simulink model "position_by_Adaptive_RBF_Attitude_by_supervised_RBFNN"  (R2015a)
settings: Solver=ode3  StartTime=0.0  StopTime=40  FixedStep=0.001  RelTol=1e-3
libraries: simulink x12, commnoisgen2 x5, dspsrcs4 x1
(part 1 of 2)
settings Model: SimulationMode=accelerator  Creator=user  LastModifiedBy=user

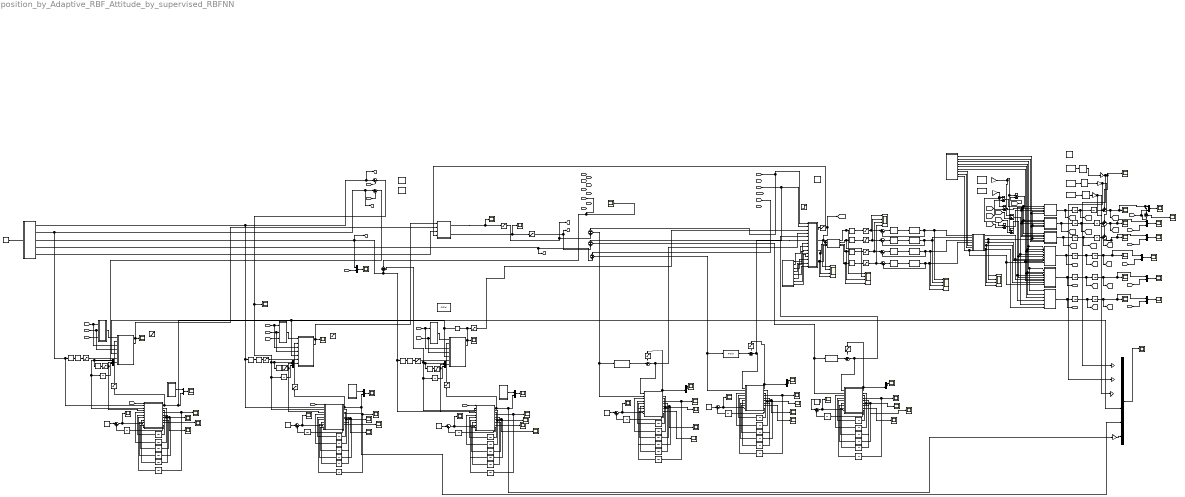
== system position_by_Adaptive_RBF_Attitude_by_supervised_RBFNN ==
  note: Linear position Adaptive RBF NN based control
  note: Attitude supervisory control based on RBF NN
  note: error of z
  note: 0.178
  note: 0.16
  note: used to extract data
  note: Adaptive RBFNN Position+ SUPERVISED RBF-PID attitude CONTROL-Final- VG results
  note: d25
  Constant{1..6} (6 alike) : Constant  Value=0
  DATA : MATLAB Function  TreatAsAtomicUnit=on
  DATA1 : MATLAB Function  TreatAsAtomicUnit=on
  Delay1 : Delay  DelayLength=1  SampleTime=0.001
  Derivative{,1..8} (9 alike) : Derivative
  Gain : Gain  Gain=0.01
  Gain1 : Gain  Gain=0.01
  Gain2 : Gain  Gain=2000
  Gain3 : Gain  Gain=2000
  Gain4 : Gain  Gain=2000
  Gain5 : Gain  Gain=0.1
  Gain6 : Gain  Gain=0.07
  Gain7 : Gain  Gain=0.07
  Gain8 : Gain  Gain=7
  Gaussian Noise Generator : commnoisgen2/Gaussian Noise Generator  m=0  d=1  s=41  Ts=0.02  frameBased=off  sampPerFrame=1  orient=off  outDataType=double
  Gaussian Noise Generator1 : commnoisgen2/Gaussian Noise Generator  m=0  d=1  s=41  Ts=0.02  frameBased=off  sampPerFrame=1  orient=off  outDataType=double
  Gaussian Noise Generator3 : commnoisgen2/Gaussian Noise Generator  m=0.3  d=1  s=41  Ts=5  frameBased=off  sampPerFrame=1  orient=off  outDataType=double
  Gaussian Noise Generator5 : commnoisgen2/Gaussian Noise Generator  m=0.3  d=1  s=41  Ts=2.5  frameBased=off  sampPerFrame=1  orient=off  outDataType=double
  Gaussian Noise Generator6 : commnoisgen2/Gaussian Noise Generator  m=0.3  d=1  s=41  Ts=3.5  frameBased=off  sampPerFrame=1  orient=on  outDataType=double
  Integrator{1..15} (15 alike) : Integrator
  MATLAB Function : MATLAB Function  TreatAsAtomicUnit=on
  MATLAB Function1 : MATLAB Function  TreatAsAtomicUnit=on
  MATLAB Function2 : MATLAB Function  TreatAsAtomicUnit=on
  MATLAB Function3 : MATLAB Function  TreatAsAtomicUnit=on
  MATLAB Function4 : MATLAB Function  TreatAsAtomicUnit=on
  MATLAB Function5 : MATLAB Function  TreatAsAtomicUnit=on
  MATLAB Function6 : MATLAB Function  TreatAsAtomicUnit=on
  MATLAB Function7 : MATLAB Function  TreatAsAtomicUnit=on
  MATLAB Function8 : MATLAB Function  TreatAsAtomicUnit=on
  Mux : Mux  Inputs=3
  Mux{1..10,12..13,15} (13 alike) : Mux  Inputs=2
  Mux11 : Mux  Inputs=3
  Mux14 : Mux  Inputs=3
  Mux16 : Mux  Inputs=6
  Omega i ^2  calc : MATLAB Function  TreatAsAtomicUnit=on
  Omegas : Scope  NumInputPorts=4
      settings: YMin=-5~-5~-5~-5  YMax=5~5~5~5  SaveName=ScopeData3
  PID Controller{,4..6} (4 alike) : simulink/Continuous/PID Controller  Controller=PID  TimeDomain=Continuous-time  SampleTime=-1  IntegratorMethod=Forward Euler  FilterMethod=Forward Euler  Form=Parallel  UseFilter=on  ControllerParametersSource=internal  P=0.696663945518539  I=69.3627675374527  D=0.000480635781112464  N=569.937710840054  InitialConditionSource=internal  InitialConditionForIntegrator=0  InitialConditionForFilter=0  ExternalReset=none  LimitOutput=off  UpperSaturationLimit=+12  LowerSaturationLimit=-12  LinearizeAsGain=on  AntiWindupMode=clamping  Kb=1  TrackingMode=off  Kt=1  PParamMin=[]  PParamMax=[]  IParamMin=[]  IParamMax=[]  DParamMin=[]  DParamMax=[]  NParamMin=[]  NParamMax=[]  KbParamMin=[]  KbParamMax=[]  KtParamMin=[]  KtParamMax=[]  POutMin=[]  POutMax=[]  IOutMin=[]  IOutMax=[]  DOutMin=[]  DOutMax=[]  NOutMin=[]  NOutMax=[]  KbOutMin=[]  KbOutMax=[]  KtOutMin=[]  KtOutMax=[]  IntegratorOutMin=[]  IntegratorOutMax=[]  FilterOutMin=[]  FilterOutMax=[]  SumOutMin=[]  SumOutMax=[]  SumI1OutMin=[]  SumI1OutMax=[]  SumI2OutMin=[]  SumI2OutMax=[]  SumI3OutMin=[]  SumI3OutMax=[]  SumDOutMin=[]  SumDOutMax=[]  SaturationOutMin=[]  SaturationOutMax=[]  IntegratorContinuousStateAttributes=''  IntegratorStateMustResolveToSignalObject=off  IntegratorRTWStateStorageClass=Auto  FilterContinuousStateAttributes=''  FilterStateMustResolveToSignalObject=off  FilterRTWStateStorageClass=Auto  DifferentiatorICPrevScaledInput=0  DifferentiatorOutMin=[]  DifferentiatorOutMax=[]
  PID Controller1 : simulink/Continuous/PID Controller  Controller=PID  TimeDomain=Continuous-time  SampleTime=-1  IntegratorMethod=Forward Euler  FilterMethod=Forward Euler  Form=Parallel  UseFilter=on  ControllerParametersSource=internal  P=4  I=2  D=5  N=476.409993785115  InitialConditionSource=internal  InitialConditionForIntegrator=0  InitialConditionForFilter=0  ExternalReset=none  LimitOutput=off  UpperSaturationLimit=inf  LowerSaturationLimit=-inf  LinearizeAsGain=on  AntiWindupMode=none  Kb=1  TrackingMode=off  Kt=1  PParamMin=[]  PParamMax=[]  IParamMin=[]  IParamMax=[]  DParamMin=[]  DParamMax=[]  NParamMin=[]  NParamMax=[]  KbParamMin=[]  KbParamMax=[]  KtParamMin=[]  KtParamMax=[]  POutMin=[]  POutMax=[]  IOutMin=[]  IOutMax=[]  DOutMin=[]  DOutMax=[]  NOutMin=[]  NOutMax=[]  KbOutMin=[]  KbOutMax=[]  KtOutMin=[]  KtOutMax=[]  IntegratorOutMin=[]  IntegratorOutMax=[]  FilterOutMin=[]  FilterOutMax=[]  SumOutMin=[]  SumOutMax=[]  SumI1OutMin=[]  SumI1OutMax=[]  SumI2OutMin=[]  SumI2OutMax=[]  SumI3OutMin=[]  SumI3OutMax=[]  SumDOutMin=[]  SumDOutMax=[]  SaturationOutMin=[]  SaturationOutMax=[]  IntegratorContinuousStateAttributes=''  IntegratorStateMustResolveToSignalObject=off  IntegratorRTWStateStorageClass=Auto  FilterContinuousStateAttributes=''  FilterStateMustResolveToSignalObject=off  FilterRTWStateStorageClass=Auto  DifferentiatorICPrevScaledInput=0  DifferentiatorOutMin=[]  DifferentiatorOutMax=[]
  PID Controller14 : simulink/Continuous/PID Controller  Controller=PID  TimeDomain=Continuous-time  SampleTime=-1  IntegratorMethod=Forward Euler  FilterMethod=Forward Euler  Form=Parallel  UseFilter=on  ControllerParametersSource=internal  P=1.8  I=0.4  D=2.4  N=100  InitialConditionSource=internal  InitialConditionForIntegrator=0  InitialConditionForFilter=0  ExternalReset=none  LimitOutput=off  UpperSaturationLimit=inf  LowerSaturationLimit=-inf  LinearizeAsGain=on  AntiWindupMode=none  Kb=1  TrackingMode=off  Kt=1  PParamMin=[]  PParamMax=[]  IParamMin=[]  IParamMax=[]  DParamMin=[]  DParamMax=[]  NParamMin=[]  NParamMax=[]  KbParamMin=[]  KbParamMax=[]  KtParamMin=[]  KtParamMax=[]  POutMin=[]  POutMax=[]  IOutMin=[]  IOutMax=[]  DOutMin=[]  DOutMax=[]  NOutMin=[]  NOutMax=[]  KbOutMin=[]  KbOutMax=[]  KtOutMin=[]  KtOutMax=[]  IntegratorOutMin=[]  IntegratorOutMax=[]  FilterOutMin=[]  FilterOutMax=[]  SumOutMin=[]  SumOutMax=[]  SumI1OutMin=[]  SumI1OutMax=[]  SumI2OutMin=[]  SumI2OutMax=[]  SumI3OutMin=[]  SumI3OutMax=[]  SumDOutMin=[]  SumDOutMax=[]  SaturationOutMin=[]  SaturationOutMax=[]  IntegratorContinuousStateAttributes=''  IntegratorStateMustResolveToSignalObject=off  IntegratorRTWStateStorageClass=Auto  FilterContinuousStateAttributes=''  FilterStateMustResolveToSignalObject=off  FilterRTWStateStorageClass=Auto  DifferentiatorICPrevScaledInput=0  DifferentiatorOutMin=[]  DifferentiatorOutMax=[]
  PID Controller15 : simulink/Continuous/PID Controller  Controller=PID  TimeDomain=Continuous-time  SampleTime=-1  IntegratorMethod=Forward Euler  FilterMethod=Forward Euler  Form=Parallel  UseFilter=on  ControllerParametersSource=internal  P=1.8  I=0.4  D=2.1  N=100  InitialConditionSource=internal  InitialConditionForIntegrator=0  InitialConditionForFilter=0  ExternalReset=none  LimitOutput=off  UpperSaturationLimit=inf  LowerSaturationLimit=-inf  LinearizeAsGain=on  AntiWindupMode=none  Kb=1  TrackingMode=off  Kt=1  PParamMin=[]  PParamMax=[]  IParamMin=[]  IParamMax=[]  DParamMin=[]  DParamMax=[]  NParamMin=[]  NParamMax=[]  KbParamMin=[]  KbParamMax=[]  KtParamMin=[]  KtParamMax=[]  POutMin=[]  POutMax=[]  IOutMin=[]  IOutMax=[]  DOutMin=[]  DOutMax=[]  NOutMin=[]  NOutMax=[]  KbOutMin=[]  KbOutMax=[]  KtOutMin=[]  KtOutMax=[]  IntegratorOutMin=[]  IntegratorOutMax=[]  FilterOutMin=[]  FilterOutMax=[]  SumOutMin=[]  SumOutMax=[]  SumI1OutMin=[]  SumI1OutMax=[]  SumI2OutMin=[]  SumI2OutMax=[]  SumI3OutMin=[]  SumI3OutMax=[]  SumDOutMin=[]  SumDOutMax=[]  SaturationOutMin=[]  SaturationOutMax=[]  IntegratorContinuousStateAttributes=''  IntegratorStateMustResolveToSignalObject=off  IntegratorRTWStateStorageClass=Auto  FilterContinuousStateAttributes=''  FilterStateMustResolveToSignalObject=off  FilterRTWStateStorageClass=Auto  DifferentiatorICPrevScaledInput=0  DifferentiatorOutMin=[]  DifferentiatorOutMax=[]
  PID Controller2 : simulink/Continuous/PID Controller  Controller=PID  TimeDomain=Continuous-time  SampleTime=-1  IntegratorMethod=Forward Euler  FilterMethod=Forward Euler  Form=Parallel  UseFilter=on  ControllerParametersSource=internal  P=4.05643234281984  I=0.70959032661118  D=4.0859309721323  N=476.409993785115  InitialConditionSource=internal  InitialConditionForIntegrator=0  InitialConditionForFilter=0  ExternalReset=none  LimitOutput=off  UpperSaturationLimit=inf  LowerSaturationLimit=-inf  LinearizeAsGain=on  AntiWindupMode=none  Kb=1  TrackingMode=off  Kt=1  PParamMin=[]  PParamMax=[]  IParamMin=[]  IParamMax=[]  DParamMin=[]  DParamMax=[]  NParamMin=[]  NParamMax=[]  KbParamMin=[]  KbParamMax=[]  KtParamMin=[]  KtParamMax=[]  POutMin=[]  POutMax=[]  IOutMin=[]  IOutMax=[]  DOutMin=[]  DOutMax=[]  NOutMin=[]  NOutMax=[]  KbOutMin=[]  KbOutMax=[]  KtOutMin=[]  KtOutMax=[]  IntegratorOutMin=[]  IntegratorOutMax=[]  FilterOutMin=[]  FilterOutMax=[]  SumOutMin=[]  SumOutMax=[]  SumI1OutMin=[]  SumI1OutMax=[]  SumI2OutMin=[]  SumI2OutMax=[]  SumI3OutMin=[]  SumI3OutMax=[]  SumDOutMin=[]  SumDOutMax=[]  SaturationOutMin=[]  SaturationOutMax=[]  IntegratorContinuousStateAttributes=''  IntegratorStateMustResolveToSignalObject=off  IntegratorRTWStateStorageClass=Auto  FilterContinuousStateAttributes=''  FilterStateMustResolveToSignalObject=off  FilterRTWStateStorageClass=Auto  DifferentiatorICPrevScaledInput=0  DifferentiatorOutMin=[]  DifferentiatorOutMax=[]
  PID Controller3 : simulink/Continuous/PID Controller  Controller=PID  TimeDomain=Continuous-time  SampleTime=-1  IntegratorMethod=Forward Euler  FilterMethod=Forward Euler  Form=Parallel  UseFilter=on  ControllerParametersSource=internal  P=11  I=0.2  D=22  N=100  InitialConditionSource=internal  InitialConditionForIntegrator=0  InitialConditionForFilter=0  ExternalReset=none  LimitOutput=off  UpperSaturationLimit=inf  LowerSaturationLimit=-inf  LinearizeAsGain=on  AntiWindupMode=none  Kb=1  TrackingMode=off  Kt=1  PParamMin=[]  PParamMax=[]  IParamMin=[]  IParamMax=[]  DParamMin=[]  DParamMax=[]  NParamMin=[]  NParamMax=[]  KbParamMin=[]  KbParamMax=[]  KtParamMin=[]  KtParamMax=[]  POutMin=[]  POutMax=[]  IOutMin=[]  IOutMax=[]  DOutMin=[]  DOutMax=[]  NOutMin=[]  NOutMax=[]  KbOutMin=[]  KbOutMax=[]  KtOutMin=[]  KtOutMax=[]  IntegratorOutMin=[]  IntegratorOutMax=[]  FilterOutMin=[]  FilterOutMax=[]  SumOutMin=[]  SumOutMax=[]  SumI1OutMin=[]  SumI1OutMax=[]  SumI2OutMin=[]  SumI2OutMax=[]  SumI3OutMin=[]  SumI3OutMax=[]  SumDOutMin=[]  SumDOutMax=[]  SaturationOutMin=[]  SaturationOutMax=[]  IntegratorContinuousStateAttributes=''  IntegratorStateMustResolveToSignalObject=off  IntegratorRTWStateStorageClass=Auto  FilterContinuousStateAttributes=''  FilterStateMustResolveToSignalObject=off  FilterRTWStateStorageClass=Auto  DifferentiatorICPrevScaledInput=0  DifferentiatorOutMin=[]  DifferentiatorOutMax=[]
  PID Controller7 : simulink/Continuous/PID Controller  Controller=PID  TimeDomain=Continuous-time  SampleTime=-1  IntegratorMethod=Forward Euler  FilterMethod=Forward Euler  Form=Parallel  UseFilter=on  ControllerParametersSource=internal  P=12  I=0.2  D=14  N=100  InitialConditionSource=internal  InitialConditionForIntegrator=0  InitialConditionForFilter=0  ExternalReset=none  LimitOutput=off  UpperSaturationLimit=inf  LowerSaturationLimit=-inf  LinearizeAsGain=on  AntiWindupMode=none  Kb=1  TrackingMode=off  Kt=1  PParamMin=[]  PParamMax=[]  IParamMin=[]  IParamMax=[]  DParamMin=[]  DParamMax=[]  NParamMin=[]  NParamMax=[]  KbParamMin=[]  KbParamMax=[]  KtParamMin=[]  KtParamMax=[]  POutMin=[]  POutMax=[]  IOutMin=[]  IOutMax=[]  DOutMin=[]  DOutMax=[]  NOutMin=[]  NOutMax=[]  KbOutMin=[]  KbOutMax=[]  KtOutMin=[]  KtOutMax=[]  IntegratorOutMin=[]  IntegratorOutMax=[]  FilterOutMin=[]  FilterOutMax=[]  SumOutMin=[]  SumOutMax=[]  SumI1OutMin=[]  SumI1OutMax=[]  SumI2OutMin=[]  SumI2OutMax=[]  SumI3OutMin=[]  SumI3OutMax=[]  SumDOutMin=[]  SumDOutMax=[]  SaturationOutMin=[]  SaturationOutMax=[]  IntegratorContinuousStateAttributes=''  IntegratorStateMustResolveToSignalObject=off  IntegratorRTWStateStorageClass=Auto  FilterContinuousStateAttributes=''  FilterStateMustResolveToSignalObject=off  FilterRTWStateStorageClass=Auto  DifferentiatorICPrevScaledInput=0  DifferentiatorOutMin=[]  DifferentiatorOutMax=[]
  PID Controller9 : simulink/Continuous/PID Controller  Controller=PID  TimeDomain=Continuous-time  SampleTime=-1  IntegratorMethod=Forward Euler  FilterMethod=Forward Euler  Form=Parallel  UseFilter=on  ControllerParametersSource=internal  P=3.4  I=0.7  D=4.3  N=100  InitialConditionSource=internal  InitialConditionForIntegrator=0  InitialConditionForFilter=0  ExternalReset=none  LimitOutput=off  UpperSaturationLimit=inf  LowerSaturationLimit=-inf  LinearizeAsGain=on  AntiWindupMode=none  Kb=1  TrackingMode=off  Kt=1  PParamMin=[]  PParamMax=[]  IParamMin=[]  IParamMax=[]  DParamMin=[]  DParamMax=[]  NParamMin=[]  NParamMax=[]  KbParamMin=[]  KbParamMax=[]  KtParamMin=[]  KtParamMax=[]  POutMin=[]  POutMax=[]  IOutMin=[]  IOutMax=[]  DOutMin=[]  DOutMax=[]  NOutMin=[]  NOutMax=[]  KbOutMin=[]  KbOutMax=[]  KtOutMin=[]  KtOutMax=[]  IntegratorOutMin=[]  IntegratorOutMax=[]  FilterOutMin=[]  FilterOutMax=[]  SumOutMin=[]  SumOutMax=[]  SumI1OutMin=[]  SumI1OutMax=[]  SumI2OutMin=[]  SumI2OutMax=[]  SumI3OutMin=[]  SumI3OutMax=[]  SumDOutMin=[]  SumDOutMax=[]  SaturationOutMin=[]  SaturationOutMax=[]  IntegratorContinuousStateAttributes=''  IntegratorStateMustResolveToSignalObject=off  IntegratorRTWStateStorageClass=Auto  FilterContinuousStateAttributes=''  FilterStateMustResolveToSignalObject=off  FilterRTWStateStorageClass=Auto  DifferentiatorICPrevScaledInput=0  DifferentiatorOutMin=[]  DifferentiatorOutMax=[]
  Phidd : MATLAB Function  TreatAsAtomicUnit=on
  Ramp1 : simulink/Sources/Ramp  slope=1  start=0  X0=0
  Random Source1 : dspsrcs4/Random Source  SrcType=Uniform  NormMethod=Ziggurat  CltLength=12  MinVal=0  MaxVal=2  MeanVal=0  VarVal=1  RepMode=Not repeatable  rawSeed=1  IsInherit=off  SampMode=Discrete  SampTime=2  SampFrame=1  DataType=Double  OutComplex=Real
  Rate Transition : RateTransition
  Rate Transition1 : RateTransition
  Rate Transition2 : RateTransition
  Saturation : Saturate  UpperLimit=3000  LowerLimit=0
  Saturation1 : Saturate  UpperLimit=3000  LowerLimit=0
  Saturation10 : Saturate  UpperLimit=150  LowerLimit=-150
  Saturation11 : Saturate  UpperLimit=200  LowerLimit=-200
  Saturation12 : Saturate  UpperLimit=100  LowerLimit=-100
  Saturation{5,13,17..19} (5 alike) : Saturate  UpperLimit=2  LowerLimit=-2
  Saturation14 : Saturate  UpperLimit=30  LowerLimit=-30
  Saturation15 : Saturate  UpperLimit=40  LowerLimit=-40
  Saturation16 : Saturate  UpperLimit=80  LowerLimit=-50
  Saturation2 : Saturate  UpperLimit=800  LowerLimit=0
  Saturation20 : Saturate  UpperLimit=30  LowerLimit=-30
  Saturation21 : Saturate  UpperLimit=400  LowerLimit=-400
  Saturation3 : Saturate  UpperLimit=800  LowerLimit=0
  Saturation4 : Saturate  UpperLimit=50  LowerLimit=1
  Saturation6 : Saturate  UpperLimit=30  LowerLimit=-30
  Saturation7 : Saturate  UpperLimit=0.4  LowerLimit=-0.4
  Saturation8 : Saturate  UpperLimit=0.4  LowerLimit=-0.41
  Saturation9 : Saturate  UpperLimit=400  LowerLimit=-400
  Scope{,1..34} (35 alike) : Scope
      Scope settings: TimeRange=10  YMin=0.00025  YMax=0.00325
      Scope10 settings: YMin=-5.5  YMax=6  SaveName=xdata
      Scope11 settings: YMin=7.989  YMax=7.9915  SaveName=zdata
      Scope12 settings: SaveName=ScopeData12
      Scope13 settings: SaveName=ScopeData20
      Scope14 settings: SaveName=ScopeData14
      Scope15 settings: SaveName=ScopeData17
      Scope16 settings: YMin=7.989  YMax=7.9915  SaveName=e1
      Scope17 settings: SaveName=ScopeData21
      Scope18 settings: SaveName=ScopeData22
      Scope19 settings: SaveName=ScopeData26
      Scope2 settings: SaveName=ScopeData8
      Scope20 settings: SaveName=ScopeData27
      Scope21 settings: SaveName=ScopeData28
      Scope22 settings: YMin=-0.55  YMax=0.45  SaveName=ScopeData11
      Scope23 settings: SaveName=ScopeData32
      Scope24 settings: SaveName=ScopeData33
      Scope25 settings: SaveName=ScopeData9
      Scope26 settings: SaveName=ScopeData35
      Scope27 settings: YMax=17  SaveName=ScopeData36
      Scope28 settings: YMin=4.98345  YMax=4.98345  SaveName=ScopeData41
      Scope29 settings: SaveName=ScopeData42
      Scope3 settings: YMin=-0.55  YMax=0.45  SaveName=ScopeData37
      Scope30 settings: SaveName=ScopeData46
      Scope31 settings: YMax=17  SaveName=ScopeData47
      Scope32 settings: YMin=-0.55  YMax=0.45  SaveName=ScopeData48
      Scope33 settings: YMin=-0.035  YMax=0.035  SaveName=xdata1
      Scope34 settings: YMin=-5.5  YMax=6  SaveName=Dist
      Scope4 settings: SaveName=ScopeData10
      Scope5 settings: YMin=-0.55  YMax=0.45  SaveName=ScopeData34
      Scope6 settings: YMin=-0.05  YMax=0.005  SaveName=phi
      Scope7 settings: YMin=-0.525  YMax=-0.275  SaveName=theta
      Scope8 settings: YMin=0  YMax=0.0175  SaveName=psi
      Scope9 settings: YMin=-1  YMax=6  SaveName=ydata
  Signed Sqrt{,1..3} (4 alike) : Sqrt  Operator=signedSqrt  SaturateOnIntegerOverflow=on
  Step1 : Step  Time=0  After=0  SampleTime=0
  Sum{,1..3,9..10} (6 alike) : Sum  Inputs=|+-
  Sum{11..12,21,24..25,31} (6 alike) : Sum  Inputs=|++
  Sum{13..14,20,22,26..27} (6 alike) : Sum  Inputs=++|
  Sum{4..8,15..19} (10 alike) : Sum  Inputs=-+
  Sum23 : Sum  Inputs=+-
  Ui : Scope  NumInputPorts=4
      settings: YMin=-5~-5~-5~-5  YMax=5~5~5~5  SaveName=ScopeData15
  Ui calculation : MATLAB Function  TreatAsAtomicUnit=on
  Unit Delay{1..42} (42 alike) : UnitDelay  SampleTime=-1
  W{,1..5} (6 alike) : Scope
      W settings: SaveName=w
      W1 settings: SaveName=ScopeData23
      W2 settings: SaveName=ScopeData29
      W3 settings: SaveName=ScopeData43
      W4 settings: SaveName=ScopeData38
      W5 settings: SaveName=ScopeData49
  X : Scope
      settings: YMin=3.81  YMax=3.95  SaveName=ScopeData6
  X1 : Scope  NumInputPorts=4
      settings: YMin=-5~-5~-5~-5  YMax=5~5~5~5  SaveName=ScopeData16
  X2 : Scope  NumInputPorts=4
      settings: YMin=-5~-5~-5~-5  YMax=5~5~5~5  SaveName=ScopeData7
  Xdd : MATLAB Function  TreatAsAtomicUnit=on
  Xdd1 : MATLAB Function  TreatAsAtomicUnit=on
  Xdd2 : MATLAB Function  TreatAsAtomicUnit=on
  Xdd3 : MATLAB Function  TreatAsAtomicUnit=on
  Xdd4 : MATLAB Function  TreatAsAtomicUnit=on
  Xdd5 : MATLAB Function  TreatAsAtomicUnit=on
  Xdd6 : MATLAB Function  TreatAsAtomicUnit=on
  Y : Scope
      settings: YMin=-0.01095  YMax=-0.0103  SaveName=ScopeData5
  Ydd : MATLAB Function  TreatAsAtomicUnit=on
  "Z " : Scope
      settings: YMin=7.615  YMax=7.6215  SaveName=ScopeData2
  Zdd : MATLAB Function  TreatAsAtomicUnit=on
  Zero-Pole{,1..3} (4 alike) : ZeroPole  Zeros=[]  Poles=[-22.5]  Gain=[509]
  angles 1 : MATLAB Function  TreatAsAtomicUnit=on
  b{,1..5} (6 alike) : Scope
      b settings: SaveName=b
      b1 settings: SaveName=ScopeData24
      b2 settings: SaveName=ScopeData30
      b3 settings: SaveName=ScopeData44
      b4 settings: SaveName=ScopeData39
      b5 settings: SaveName=ScopeData50
  c{,1..5} (6 alike) : Scope
      c settings: SaveName=c
      c1 settings: SaveName=ScopeData25
      c2 settings: SaveName=ScopeData31
      c3 settings: SaveName=ScopeData45
      c4 settings: SaveName=ScopeData40
      c5 settings: SaveName=ScopeData51
  "hjsdfd " : MATLAB Function  TreatAsAtomicUnit=on
  ksi : Scope
      settings: SaveName=ksiangle
  ksidd : MATLAB Function  TreatAsAtomicUnit=on
  omegas2 : Scope  NumInputPorts=4
      settings: YMin=-5~-5~-5~-5  YMax=5~5~5~5  SaveName=ScopeData4
  phi : Scope
      settings: SaveName=phiangle
  recalc of Ui real : MATLAB Function  TreatAsAtomicUnit=on
  theta : Scope
      settings: SaveName=thetaangle
  thetadd : MATLAB Function  TreatAsAtomicUnit=on
  Out2 : Outport
  Out3 : Outport  Port=2
  Out4 : Outport  Port=3
  wires:
  angles 1/1(phitrk) -> Saturation7/1, Scope/1
  angles 1/2(thetatrk) -> Scope1/1, Saturation8/1
  Zero-Pole/1 -> Sum/2, X1/1, recalc of Ui real/1(om1)
  Sum/1 -> PID Controller/1
  Saturation/1 -> omegas2/1, Sum/1
  PID Controller/1 -> Zero-Pole/1
  Zero-Pole1/1 -> Sum1/2, X1/2, recalc of Ui real/2(om2)
  Sum1/1 -> PID Controller4/1
  Saturation1/1 -> omegas2/2, Sum1/1
  PID Controller4/1 -> Zero-Pole1/1
  Zero-Pole2/1 -> Sum2/2, X1/3, recalc of Ui real/3(om3)
  Sum2/1 -> PID Controller5/1
  Saturation2/1 -> omegas2/3, Sum2/1
  PID Controller5/1 -> Zero-Pole2/1
  Zero-Pole3/1 -> Sum3/2, X1/4, recalc of Ui real/4(om4)
  Sum3/1 -> PID Controller6/1
  Saturation3/1 -> omegas2/4, Sum3/1
  PID Controller6/1 -> Zero-Pole3/1
  Signed Sqrt/1 -> Saturation/1
  Signed Sqrt1/1 -> Saturation1/1
  Signed Sqrt2/1 -> Saturation2/1
  Signed Sqrt3/1 -> Saturation3/1
  Saturation4/1 -> angles 1/4(U1), Ui/1, Omega i ^2  calc/1(u1), [U1]
  Ui calculation/2(u2) -> Ui/2, Omega i ^2  calc/2(u2)
  Ui calculation/4(u4) -> Ui/4, Omega i ^2  calc/4(u4)
  Xdd/1(Xdd) -> [Xdd], Integrator1/1
  Ydd/1(Ydd) -> [Ydd], Integrator3/1
  Zdd/1(Zdd) -> [zdd], Integrator5/1
  Phidd/1(phidd) -> Out2/1, Integrator7/1
  Integrator7/1 -> [phid], Integrator8/1
  thetadd/1(thetadd) -> Out3/1, Integrator9/1
  Integrator9/1 -> [thetad], Integrator10/1
  ksidd/1(ksidd) -> Out4/1, Integrator11/1
  Integrator11/1 -> [ksid], Integrator12/1
  Integrator8/1 -> Mux2/1, phi/1, [phi]
  DATA/1(m) -> Zdd/5(m), Ydd/5(m), Xdd/5(m)
  DATA/2(g) -> Zdd/6(g)
  DATA/3(Ixx) -> ksidd/1(Ixx), thetadd/1(Ixx), Phidd/1(Ixx)
  DATA/4(Iyy) -> Phidd/2(Iyy), ksidd/2(Iyy), thetadd/2(Iyy)
  DATA/5(Izz) -> thetadd/3(Izz), ksidd/3(Izz), Phidd/3(Izz)
  DATA/6(J) -> thetadd/7(J), Phidd/7(J)
  Sum15/1 -> Zdd/1(phi), Ydd/1(phi), Xdd/1(phi)
  Sum4/1 -> Zdd/2(theta), Ydd/2(theta), Xdd/2(theta)
  Sum16/1 -> Ydd/3(ksi), Zdd/3(ksi), Xdd/3(ksi)
  Sum18/1 -> Phidd/4(thetad), ksidd/5(thetad)
  Sum19/1 -> Phidd/5(ksid), thetadd/5(ksid)
  Sum17/1 -> ksidd/4(phid), thetadd/4(phid)
  recalc of Ui real/1(omega) -> thetadd/6(omega), Phidd/6(omega)
  DATA/7(b) -> recalc of Ui real/5(b)
  DATA/8(d) -> recalc of Ui real/6(d)
  DATA1/1(m) -> Ui calculation/7(m)
  DATA1/2(g) -> Ui calculation/8(g)
  DATA1/6(b) -> Ui calculation/9(b)
  DATA1/7(d) -> Ui calculation/10(d)
  DATA1/8(l) -> Ui calculation/11(l)
  DATA1/3(Ixx) -> Ui calculation/12(Ixx)
  DATA1/4(Iyy) -> Ui calculation/13(Iyy)
  DATA1/5(Izz) -> Ui calculation/14(Izz)
  recalc of Ui real/5(u4) -> X2/4, ksidd/6(u4)
  recalc of Ui real/4(u3) -> X2/3, thetadd/8(u3)
  recalc of Ui real/3(u2) -> X2/2, Phidd/8(u2)
  Ui calculation/3(u3) -> Ui/3, Omega i ^2  calc/3(u3)
  Omega i ^2  calc/1(om1) -> Omegas/1, Signed Sqrt/1
  Omega i ^2  calc/2(om2) -> Omegas/2, Signed Sqrt1/1
  Omega i ^2  calc/3(om3) -> Omegas/3, Signed Sqrt2/1
  Omega i ^2  calc/4(om4) -> Omegas/4, Signed Sqrt3/1
  Gain1/1 -> Sum16/1, Sum4/1, Sum15/1
  [phi] -> Sum15/2
  [theta] -> Sum4/2
  [ksi] -> Sum16/2
  Gain/1 -> Sum19/1, Sum17/1, Sum18/1
  [phid] -> Sum17/2
  [thetad] -> Sum18/2
  [ksid] -> Sum19/2
  recalc of Ui real/2(u1) -> X2/1, Zdd/4(u1), Ydd/4(u1), Xdd/4(u1)
  Integrator5/1 -> [zd], Integrator6/1
  Integrator3/1 -> [Yd], Integrator4/1
  Integrator1/1 -> [Xd], Integrator2/1
  DATA/9(l) -> Phidd/9(l), thetadd/9(l), recalc of Ui real/7(l)
  [Z] -> Sum5/1, Scope2/1
  [phi] -> Ui calculation/1(phi), Sum7/1
  [theta] -> Ui calculation/2(theta), Sum8/1
  [ksi] -> Sum6/1
  Saturation7/1 -> [phidesired], Sum7/2
  "hjsdfd "/5(m) -> angles 1/3(m)
  Ui calculation/1(u1) -> Saturation4/1
  [Z] -> Mux1/2
  Mux1/1 -> Scope4/1
  [phidesired] -> Mux2/2
  Mux2/1 -> Scope6/1
  Integrator10/1 -> [theta], Mux3/1, theta/1
  [thetadesired] -> Mux3/2
  Mux3/1 -> Scope7/1
  Integrator12/1 -> [ksi], Mux4/1, ksi/1
  [Ksidesired] -> Mux4/2
  Mux4/1 -> Scope8/1
  "hjsdfd "/4(ksides) -> [Ksidesired], Sum6/2
  [X] -> Sum10/2
  [Y] -> Sum9/2
  Sum14/1 -> [Y], Mux5/1, Y/1
  [YYY] -> Mux5/2
  Mux5/1 -> Scope9/1
  Sum13/1 -> [X], Sum23/1, Mux6/1, X/1
  [XXX] -> Sum23/2, Mux6/2
  Mux6/1 -> Scope10/1
  Sum20/1 -> Mux7/1, "Z "/1, [Z]
  [ZZZ] -> Mux7/2
  Mux7/1 -> Scope11/1
  MATLAB Function6/1(U1) -> Scope27/1, angles 1/1(Xdes)
  Saturation8/1 -> [thetadesired], Sum8/2
  Integrator2/1 -> Sum13/2
  Integrator4/1 -> Sum14/2
  Integrator6/1 -> Sum20/2
  Sum22/1 -> MATLAB Function/1(y), Ui calculation/4(phidd)
  Mux8/1 -> Scope12/1
  MATLAB Function/3(w2) -> Unit Delay2/1
  MATLAB Function/2(w1) -> Unit Delay1/1, W/1
  Unit Delay2/1 -> MATLAB Function/4(w_2)
  Unit Delay1/1 -> MATLAB Function/3(w_1)
  Sum7/1 -> MATLAB Function/2(u), PID Controller3/1
  MATLAB Function/8(o) -> Scope14/1
  Constant1/1 -> Sum21/1
  Sum21/1 -> Scope15/1, MATLAB Function/9(i)
  MATLAB Function/9(ii) -> Unit Delay3/1
  Unit Delay3/1 -> Sum21/2
  MATLAB Function/7(c2) -> Unit Delay4/1
  MATLAB Function/6(c1) -> c/1, Unit Delay5/1
  MATLAB Function/5(b2) -> Unit Delay6/1
  Unit Delay4/1 -> MATLAB Function/8(c_2)
  Unit Delay5/1 -> MATLAB Function/7(c_1)
  Unit Delay6/1 -> MATLAB Function/6(b_2)
  Unit Delay7/1 -> MATLAB Function/5(b_1)
  MATLAB Function/4(b1) -> Unit Delay7/1, b/1
  MATLAB Function/1(ym) -> Mux8/2, Saturation10/1
  Saturation10/1 -> ?
  PID Controller3/1 -> Sum22/2
  Sum23/1 -> Scope16/1
  Sum26/1 -> MATLAB Function1/1(y), Ui calculation/6(ksidd)
  Mux9/1 -> Scope13/1
  MATLAB Function1/3(w2) -> Unit Delay9/1
  MATLAB Function1/2(w1) -> Unit Delay8/1, W1/1
  Unit Delay9/1 -> MATLAB Function1/4(w_2)
  Unit Delay8/1 -> MATLAB Function1/3(w_1)
  Sum6/1 -> MATLAB Function1/2(u), PID Controller2/1
  MATLAB Function1/8(o) -> Scope17/1
  Constant2/1 -> Sum24/1
  Sum24/1 -> Scope18/1, MATLAB Function1/9(i)
  MATLAB Function1/9(ii) -> Unit Delay10/1
  Unit Delay10/1 -> Sum24/2
  MATLAB Function1/7(c2) -> Unit Delay11/1
  MATLAB Function1/6(c1) -> c1/1, Unit Delay12/1
  MATLAB Function1/5(b2) -> Unit Delay13/1
  Unit Delay11/1 -> MATLAB Function1/8(c_2)
  Unit Delay12/1 -> MATLAB Function1/7(c_1)
  Unit Delay13/1 -> MATLAB Function1/6(b_2)
  Unit Delay14/1 -> MATLAB Function1/5(b_1)
  MATLAB Function1/4(b1) -> Unit Delay14/1, b1/1
  MATLAB Function1/1(ym) -> Saturation11/1, Mux9/2
  Sum27/1 -> MATLAB Function2/1(y), Ui calculation/5(thetadd)
  Mux10/1 -> Scope19/1
  MATLAB Function2/3(w2) -> Unit Delay21/1
  MATLAB Function2/2(w1) -> Unit Delay20/1, W2/1
  Unit Delay21/1 -> MATLAB Function2/4(w_2)
  Unit Delay20/1 -> MATLAB Function2/3(w_1)
  Sum8/1 -> MATLAB Function2/2(u), PID Controller7/1
  MATLAB Function2/8(o) -> Scope20/1
  Constant3/1 -> Sum25/1
  Sum25/1 -> Scope21/1, MATLAB Function2/9(i)
  MATLAB Function2/9(ii) -> Unit Delay15/1
  Unit Delay15/1 -> Sum25/2
  MATLAB Function2/7(c2) -> Unit Delay16/1
  MATLAB Function2/6(c1) -> c2/1, Unit Delay17/1
  MATLAB Function2/5(b2) -> Unit Delay18/1
  Unit Delay16/1 -> MATLAB Function2/8(c_2)
  Unit Delay17/1 -> MATLAB Function2/7(c_1)
  Unit Delay18/1 -> MATLAB Function2/6(b_2)
  Unit Delay19/1 -> MATLAB Function2/5(b_1)
  MATLAB Function2/4(b1) -> Unit Delay19/1, b2/1
  MATLAB Function2/1(ym) -> Saturation12/1, Mux10/2
  Saturation11/1 -> ?
  PID Controller2/1 -> Sum26/2
  Saturation12/1 -> ?
  PID Controller7/1 -> Sum27/2
  Ramp1/1 -> "hjsdfd "/1(t)
  Derivative/1 -> Derivative1/1
  Derivative1/1 -> Saturation13/1
  Saturation13/1 -> MATLAB Function4/6(ydd)
  Mux/1 -> MATLAB Function4/7(E)
  Derivative2/1 -> Saturation14/1
  Saturation14/1 -> Mux/2, MATLAB Function3/4(e_d)
  MATLAB Function4/1(U1) -> Saturation15/1, Delay1/1, Scope5/1
  Sum5/1 -> MATLAB Function3/3(e), Integrator15/1, Mux/1, Derivative2/1
  Xdd2/1(G) -> MATLAB Function4/1(G)
  Integrator15/1 -> Mux/3
  Saturation15/1 -> Ui calculation/3(zdd)
  Mux13/1 -> Scope22/1
  MATLAB Function3/3(w2) -> Unit Delay23/1
  MATLAB Function3/2(w1) -> Unit Delay22/1, W3/1
  Unit Delay23/1 -> MATLAB Function3/6(w_2)
  Unit Delay22/1 -> MATLAB Function3/5(w_1)
  MATLAB Function3/8(o) -> Scope23/1
  Constant4/1 -> Sum31/1
  Sum31/1 -> Scope24/1, MATLAB Function3/11(i)
  MATLAB Function3/9(ii) -> Unit Delay24/1
  Unit Delay24/1 -> Sum31/2
  MATLAB Function3/7(c2) -> Unit Delay25/1
  MATLAB Function3/6(c1) -> c3/1, Unit Delay26/1
  MATLAB Function3/5(b2) -> Unit Delay27/1
  Unit Delay25/1 -> MATLAB Function3/10(c_2)
  Unit Delay26/1 -> MATLAB Function3/9(c_1)
  Unit Delay27/1 -> MATLAB Function3/8(b_2)
  Unit Delay28/1 -> MATLAB Function3/7(b_1)
  MATLAB Function3/4(b1) -> Unit Delay28/1, b3/1
  Xdd3/1(fest) -> Mux13/1
  Saturation16/1 -> MATLAB Function4/2(F_est)
  "hjsdfd "/3(Zdes) -> Mux1/1, MATLAB Function3/2(u), Derivative/1, Sum5/2, [ZZZ]
  [Z] -> MATLAB Function3/1(y)
  [phi] -> MATLAB Function4/3(phi), Xdd2/1(phi)
  [theta] -> MATLAB Function4/4(theta), Xdd2/2(theta)
  Derivative3/1 -> Derivative4/1
  Derivative4/1 -> Saturation5/1
  Saturation5/1 -> MATLAB Function6/6(ydd)
  Mux11/1 -> MATLAB Function6/7(E)
  Derivative5/1 -> Saturation6/1
  Saturation6/1 -> Mux11/2, MATLAB Function5/4(e_d)
  Sum10/1 -> Scope28/1, Mux11/1, Derivative5/1, MATLAB Function5/3(e), Integrator13/1
  Xdd1/1(G) -> MATLAB Function6/1(G)
  Integrator13/1 -> Mux11/3
  Mux12/1 -> Scope3/1
  MATLAB Function5/3(w2) -> Unit Delay30/1
  MATLAB Function5/2(w1) -> Unit Delay29/1, W4/1
  Unit Delay30/1 -> MATLAB Function5/6(w_2)
  Unit Delay29/1 -> MATLAB Function5/5(w_1)
  MATLAB Function5/8(o) -> Scope25/1
  Constant5/1 -> Sum11/1
  Sum11/1 -> Scope26/1, MATLAB Function5/11(i)
  MATLAB Function5/9(ii) -> Unit Delay31/1
  Unit Delay31/1 -> Sum11/2
  MATLAB Function5/7(c2) -> Unit Delay32/1
  MATLAB Function5/6(c1) -> c4/1, Unit Delay33/1
  MATLAB Function5/5(b2) -> Unit Delay34/1
  Unit Delay32/1 -> MATLAB Function5/10(c_2)
  Unit Delay33/1 -> MATLAB Function5/9(c_1)
  Unit Delay34/1 -> MATLAB Function5/8(b_2)
  Unit Delay35/1 -> MATLAB Function5/7(b_1)
  MATLAB Function5/4(b1) -> Unit Delay35/1, b4/1
  Xdd4/1(fest) -> Mux12/1
  "hjsdfd "/1(Xdes) -> [XXX], Sum10/1, Derivative3/1, MATLAB Function5/2(u)
  [X] -> MATLAB Function5/1(y)
  [phi] -> MATLAB Function6/3(phi), Xdd1/1(phi)
  [theta] -> MATLAB Function6/4(theta), Xdd1/2(theta)
  [ksi] -> Xdd1/3(ksi)
  Saturation17/1 -> MATLAB Function6/2(F_est)
  MATLAB Function8/1(U1) -> angles 1/2(Ydes), Scope31/1
  Derivative6/1 -> Derivative7/1
  Derivative7/1 -> Saturation19/1
  Saturation19/1 -> MATLAB Function8/6(ydd)
  Mux14/1 -> MATLAB Function8/7(E)
  Derivative8/1 -> Saturation20/1
  Saturation20/1 -> Mux14/2, MATLAB Function7/4(e_d)
  Sum9/1 -> MATLAB Function7/3(e), Integrator14/1, Mux14/1, Derivative8/1
  Xdd5/1(G) -> MATLAB Function8/1(G)
  Integrator14/1 -> Mux14/3
  Mux15/1 -> Scope32/1
  MATLAB Function7/3(w2) -> Unit Delay37/1
  MATLAB Function7/2(w1) -> Unit Delay36/1, W5/1
  Unit Delay37/1 -> MATLAB Function7/6(w_2)
  Unit Delay36/1 -> MATLAB Function7/5(w_1)
  MATLAB Function7/8(o) -> Scope29/1
  Constant6/1 -> Sum12/1
  Sum12/1 -> Scope30/1, MATLAB Function7/11(i)
  MATLAB Function7/9(ii) -> Unit Delay38/1
  Unit Delay38/1 -> Sum12/2
  MATLAB Function7/7(c2) -> Unit Delay39/1
  MATLAB Function7/6(c1) -> c5/1, Unit Delay40/1
  MATLAB Function7/5(b2) -> Unit Delay41/1
  Unit Delay39/1 -> MATLAB Function7/10(c_2)
  Unit Delay40/1 -> MATLAB Function7/9(c_1)
  Unit Delay41/1 -> MATLAB Function7/8(b_2)
  Unit Delay42/1 -> MATLAB Function7/7(b_1)
  MATLAB Function7/4(b1) -> Unit Delay42/1, b5/1
  Xdd6/1(fest) -> Mux15/1
  "hjsdfd "/2(Ydes) -> Sum9/1, [YYY], Derivative6/1, MATLAB Function7/2(u)
  Delay1/1 -> MATLAB Function8/5(zdd), MATLAB Function6/5(zdd), MATLAB Function4/5(zdd)
  [X] -> MATLAB Function7/1(y)
  [phi] -> MATLAB Function8/3(phi), Xdd5/1(phi)
  [theta] -> MATLAB Function8/4(theta), Xdd5/2(theta)
  [ksi] -> Xdd5/3(ksi)
  Saturation18/1 -> MATLAB Function8/2(F_est)
  Gaussian Noise Generator6/1 -> Rate Transition/1
  Gaussian Noise Generator5/1 -> Rate Transition1/1
  Gaussian Noise Generator3/1 -> Rate Transition2/1
  Rate Transition/1 -> Gain7/1
  Rate Transition1/1 -> Gain6/1
  Rate Transition2/1 -> Gain5/1
  Mux16/1 -> Scope34/1
  MATLAB Function3/1(ym) -> Saturation16/1, Gain8/1, Mux13/2
  MATLAB Function5/1(ym) -> Saturation17/1, Mux12/2, Mux16/5
  MATLAB Function7/1(ym) -> Saturation18/1, Mux16/4, Mux15/2
  Gain7/1 -> Gain2/1, Sum13/1, Scope33/1
  Gain6/1 -> Gain3/1, Sum14/1
  Gain5/1 -> Gain4/1, Sum20/1
  Gain8/1 -> Mux16/6

== matlab function position_by_Adaptive_RBF_Attitude_by_supervised_RBFNN/Ydd ==
  data: phi input; Ydd output; theta input; ksi input; u1 input; m input
function Ydd = fcn(phi,theta, ksi,u1,m)
m=1;

Ydd=(-cos(ksi)*sin(phi)+sin(ksi)*sin(theta)*cos(phi))*u1/m;

== matlab function position_by_Adaptive_RBF_Attitude_by_supervised_RBFNN/Zdd ==
  data: phi input; Zdd output; theta input; ksi input; u1 input; m input; g input
function Zdd = fcn(phi,theta, ksi,u1,m,g)
m=1;
g=9.81;

Zdd=-g+(cos(theta)*cos(phi))*u1/m;

== matlab function position_by_Adaptive_RBF_Attitude_by_supervised_RBFNN/DATA ==
  data: m output; g output; Ixx output; Iyy output; Izz output; J output; b output; d output; l output
function [m,g,Ixx,Iyy,Izz,J,b,d,l] = fcn
m=1;
g=9.81;

Ixx=1*0.008;
Iyy=1*0.008;
Izz=1*0.015;
b=0.0001;
d=0.000001;
l=0.25;
J=0.0001;

== matlab function position_by_Adaptive_RBF_Attitude_by_supervised_RBFNN/Phidd ==
  data: Ixx input; Iyy input; phidd output; Izz input; thetad input; ksid input; omega input; J input; u2 input; l input
function phidd = fcn(Ixx,Iyy,Izz,thetad, ksid,omega,J,u2,l)


phidd=1/Ixx*((Iyy-Izz)*thetad*ksid-J*thetad*omega+l*u2);

== matlab function position_by_Adaptive_RBF_Attitude_by_supervised_RBFNN/thetadd ==
  data: Ixx input; Iyy input; thetadd output; Izz input; phid input; ksid input; omega input; J input; u3 input; l input
function thetadd = fcn(Ixx,Iyy,Izz,phid, ksid,omega,J,u3,l)


thetadd=1/Iyy*((Izz-Ixx)*phid*ksid+J*phid*omega+l*u3);

== matlab function position_by_Adaptive_RBF_Attitude_by_supervised_RBFNN/ksidd ==
  data: Ixx input; Iyy input; ksidd output; Izz input; phid input; thetad input; u4 input
function ksidd = fcn(Ixx,Iyy,Izz,phid, thetad,u4)


ksidd=1/Izz*((Ixx-Iyy)*phid*thetad+u4);

== matlab function position_by_Adaptive_RBF_Attitude_by_supervised_RBFNN/Omega i ^2  calc ==
  data: u1 input; om1 output; u2 input; u3 input; u4 input; om2 output; om3 output; om4 output
function [om1,om2,om3,om4] = fcn(u1,u2,u3,u4)
%#codegen
b=0.0001;
d=0.000001;
l=0.25;
A=[ 1/(4*b),0, -1/(2*b*l), -1/(4*d);1/(4*b), -1/(2*b*l),0,  1/(4*d); 1/(4*b),  0,  1/(2*b*l), -1/(4*d);1/(4*b),1/(2*b*l), 0,  1/(4*d)];
B=A*[u1;u2;u3;u4];
%[om1;om2;om3;om4]
om1= B(1);
om2=B(2);
om3=B(3);
om4=B(4);

== matlab function position_by_Adaptive_RBF_Attitude_by_supervised_RBFNN/Ui calculation ==
  data: phi input; theta input; zdd input; u1 output; phidd input; thetadd input; ksidd input; u2 output; u3 output; u4 output; m input; g input; b input; d input; l input; Ixx input; Iyy input; Izz input
function [u1,u2,u3,u4] = fcn(phi, theta ,zdd, phidd, thetadd,ksidd,m,g,b,d,l,Ixx,Iyy,Izz )
%#codegen
u1=0;
u2=0;
u3=0;
u4=0;
u1= (zdd+g)*m/(cos(theta)*cos(phi));
u2= phidd*Ixx;
u3= thetadd*Iyy;
u4= ksidd*Izz;
b;
d;
l;
m;
g;

% if theta ==pi/2
%     u1=100;
% else 
%     if phi==pi/2
%         u1=100;
%     else
%             
% u1= (zdd+g)*m/(cos(theta)*cos(phi));
% u2= phidd*Ixx;
% u3= thetadd*Iyy;
% u4= ksidd*Izz;
% b;
% d;
% l;
% m;
% g;
% 
%     end
% end

== matlab function position_by_Adaptive_RBF_Attitude_by_supervised_RBFNN/Xdd ==
  data: phi input; Xdd output; theta input; ksi input; u1 input; m input
function Xdd = fcn(phi,theta, ksi,u1,m)


Xdd=(sin(ksi)*sin(phi)+cos(ksi)*sin(theta)*cos(phi))*u1/m;

== matlab function position_by_Adaptive_RBF_Attitude_by_supervised_RBFNN/recalc of Ui real ==
  data: om1 input; omega output; om2 input; om3 input; om4 input; b input; d input; l input; u1 output; u2 output; u3 output; u4 output
function [omega, u1,u2,u3,u4] = fcn(om1,om2,om3,om4,b,d,l)


omega=-om1+om2-om3+om4;
u1=b*(om1^2+om2^2+om3^2+om4^2);
u2=l*b*(om4^2-om2^2);
u3=l*b*(om3^2-om1^2);
u4=d*(om4^2+om2^2-om1^2-om3^2);

== matlab function position_by_Adaptive_RBF_Attitude_by_supervised_RBFNN/DATA1 ==
  data: m output; g output; Ixx output; Iyy output; Izz output; b output; d output; l output
function [m,g,Ixx,Iyy,Izz,b,d,l] = fcn
m=1;
g=9.81;

Ixx=1*0.008;
Iyy=1*0.008;
Izz=1*0.015;
b=0.0001;
d=0.000001;
l=0.25;
%J=0.0001;

== matlab function position_by_Adaptive_RBF_Attitude_by_supervised_RBFNN/MATLAB Function ==
  data: y input; u input; ym output; w_1 input; w_2 input; b_1 input; b_2 input; c_1 input; c_2 input; w1 output; w2 output; b1 output; b2 output; c1 output; c2 output; o output; i input; ii output
function [ym,w1,w2,b1,b2,c1,c2,o,ii] =System(y,u,w_1,w_2,b_1,b_2,c_1,c_2,i)
alfa=0.001;
xite=0.3;
eta =0.0000005;
gamma=0.00000001;

% alfa=0.001;
% xite=0.05;
% eta =0.005;
% gamma=0.0001;


w_1=w_1+zeros(5,1);
w_2=w_2+zeros(5,1);
b_1=b_1+zeros(5,1);
b_2=b_2+zeros(5,1);
c_1=c_1+zeros(5,1);
c_2=c_2+zeros(5,1);
if i == 0
    w=ones(5,1);
    w_1=ones(5,1);
    w_2=ones(5,1)/2;
    b=ones(5,1);
    b=[0.2; 0.2; 0.2; 0.2 ;0.2]*3; %bj
    b_1=b;
    b_2=b/2;
    c=ones(5,1);
    c=[-1.2; -0.5; 0; 0.5 ;1.2]; %cij
    c_1=c;
    c_2=c;
    
      
end

w=w_1;
w1=zeros(5,1);
w2=zeros(5,1);
b=b_1;
b1=zeros(5,1);
b2=zeros(5,1);
c=c_1;
c1=zeros(5,1);
c2=zeros(5,1);
x=u; %Input Layer
h=zeros(5,1); %hj
w=w_1;
for j=1:1:5
h(j)=exp(-norm(x-c(j))^2/(2*b(j)^2)); %Hidden Layer
end
ym=w'*h; %Output Layer

d_w=0*w;
d_w=(xite*(y-ym))*h;
w = w + d_w +alfa*(w_1 - w_2);
w2 = w_1;
w1=w;

d_b=0*b;
for k=1:5
d_b(k)=(eta*(y-ym))*w(k)*h(k)*(x-c(k))^2/b(k)^3;
end
b = b + d_b +gamma*(b_1 - b_2);

for k=1:5
if b(k)<= 0
    b(k)=0.1;
end
    
end
b2 = b_1;
b1=b;


d_c=0*c;
for k=1:5
d_c(k)=(eta*(y-ym))*w(k)*(x-c(k))/b(k)^2;
end
c = c + d_c +gamma*(c_1 - c_2);
c2 = c_1;
c1=c;

o=u;
ii=zeros(1);
ii=i+5;

== matlab function position_by_Adaptive_RBF_Attitude_by_supervised_RBFNN/hjsdfd  ==
  data: t input; Xdes output; Ydes output; Zdes output; ksides output; m output
function [Xdes,Ydes,Zdes,ksides,m] = fcn(t)

A=5;a=5;
B=10;b=4;
C=8;c=5;
Xdes=A*cos(a*0.070*t);
Ydes=A*sin(a*0.07*t);
%Zdes=C*(1-exp(-2*0.070*t));
%#codegen
m=1;
%ksides=0.2*cos(0.1*time)-0.32*sin(0.2*time);
ksides=0;
%plot3(Xdes,Ydes,Zdes,'*')
%hold on
%grid on
Zdes=t;
%Xdes=(5+sin(0.3*Zdes))*sin (2*pi*t/5);
%Ydes=(7+cos(0.3*Zdes))*cos (2*pi*t/5);

== matlab function position_by_Adaptive_RBF_Attitude_by_supervised_RBFNN/angles 1 ==
  data: Xdes input; phitrk output; Ydes input; m input; U1 input; thetatrk output
function [phitrk,thetatrk]  = fcn(Xdes,Ydes, m,U1)
%#codegen
if U1<=5
    phitrk=0;
else
    if (abs(Ydes*m/U1) >= 0.3)
        phitrk= -sign(Ydes*m/U1)*pi/10;
    else
    phitrk=-asin(Ydes*m/U1);
    end
end
%%%%%%%%%%%%%%%%%%
if U1<=5
    thetatrk=0;
elseif (abs( Xdes*m/(U1*cos(phitrk)) ) >= 0.3 )
        thetatrk = sign( Xdes*m/(U1*cos(phitrk)) )*pi/10 ;
    else
    thetatrk=asin(Xdes*m/(U1*cos(phitrk)) );
end

    
%%%%%%%%%%%%
if phitrk > pi/3
    phitrk=pi/3;
end
if phitrk < -pi/3
    phitrk=-pi/3;
end
%%%%%%%%%%%%%%%
if thetatrk > pi/3
    thetatrk=pi/3;
end
if thetatrk < -pi/3
    thetatrk=-pi/3;
end

== matlab function position_by_Adaptive_RBF_Attitude_by_supervised_RBFNN/MATLAB Function1 ==
  data: y input; u input; ym output; w_1 input; w_2 input; b_1 input; b_2 input; c_1 input; c_2 input; w1 output; w2 output; b1 output; b2 output; c1 output; c2 output; o output; i input; ii output
function [ym,w1,w2,b1,b2,c1,c2,o,ii] =System(y,u,w_1,w_2,b_1,b_2,c_1,c_2,i)
alfa=0.001;
xite=0.2;
eta =0.000005;
gamma=0.0000001;

% alfa=0.001;
% xite=0.05;
% eta =0.005;
% gamma=0.0001;


w_1=w_1+zeros(5,1);
w_2=w_2+zeros(5,1);
b_1=b_1+zeros(5,1);
b_2=b_2+zeros(5,1);
c_1=c_1+zeros(5,1);
c_2=c_2+zeros(5,1);
if i == 0
    w=ones(5,1);
    w_1=ones(5,1);
    w_2=ones(5,1)/2;
    b=ones(5,1);
    b=[0.2; 0.2; 0.2; 0.2 ;0.2]*3; %bj
    b_1=b;
    b_2=b/2;
    c=ones(5,1);
    c=[-1.2; -0.5; 0; 0.5 ;1.2]; %cij
    c_1=c;
    c_2=c;
    
      
end

w=w_1;
w1=zeros(5,1);
w2=zeros(5,1);
b=b_1;
b1=zeros(5,1);
b2=zeros(5,1);
c=c_1;
c1=zeros(5,1);
c2=zeros(5,1);
x=u; %Input Layer
h=zeros(5,1); %hj
w=w_1;
for j=1:1:5
h(j)=exp(-norm(x-c(j))^2/(2*b(j)^2)); %Hidden Layer
end
ym=w'*h; %Output Layer

d_w=0*w;
d_w=(xite*(y-ym))*h;
w = w + d_w +alfa*(w_1 - w_2);
w2 = w_1;
w1=w;

d_b=0*b;
for k=1:5
d_b(k)=(eta*(y-ym))*w(k)*h(k)*(x-c(k))^2/b(k)^3;
end
b = b + d_b +gamma*(b_1 - b_2);

for k=1:5
if b(k)<= 0
    b(k)=0.1;
end
    
end
b2 = b_1;
b1=b;


d_c=0*c;
for k=1:5
d_c(k)=(eta*(y-ym))*w(k)*(x-c(k))/b(k)^2;
end
c = c + d_c +gamma*(c_1 - c_2);
c2 = c_1;
c1=c;

o=u;
ii=zeros(1);
ii=i+5;

== matlab function position_by_Adaptive_RBF_Attitude_by_supervised_RBFNN/MATLAB Function2 ==
  data: y input; u input; ym output; w_1 input; w_2 input; b_1 input; b_2 input; c_1 input; c_2 input; w1 output; w2 output; b1 output; b2 output; c1 output; c2 output; o output; i input; ii output
function [ym,w1,w2,b1,b2,c1,c2,o,ii] =System(y,u,w_1,w_2,b_1,b_2,c_1,c_2,i)
alfa=0.05;
xite=0.07;
eta =0.000005;
gamma=0.0000001;

% alfa=0.001;
% xite=0.05;
% eta =0.005;
% gamma=0.0001;


w_1=w_1+zeros(5,1);
w_2=w_2+zeros(5,1);
b_1=b_1+zeros(5,1);
b_2=b_2+zeros(5,1);
c_1=c_1+zeros(5,1);
c_2=c_2+zeros(5,1);
if i == 0
    w=ones(5,1);
    w_1=ones(5,1);
    w_2=ones(5,1)/2;
    b=ones(5,1);
    b=[0.2; 0.2; 0.2; 0.2 ;0.2]*3; %bj
    b_1=b;
    b_2=b/2;
    c=ones(5,1);
    c=[-1.2; -0.5; 0; 0.5 ;1.2]; %cij
    c_1=c;
    c_2=c;
    
      
end

w=w_1;
w1=zeros(5,1);
w2=zeros(5,1);
b=b_1;
b1=zeros(5,1);
b2=zeros(5,1);
c=c_1;
c1=zeros(5,1);
c2=zeros(5,1);
x=u; %Input Layer
h=zeros(5,1); %hj
w=w_1;
for j=1:1:5
h(j)=exp(-norm(x-c(j))^2/(2*b(j)^2)); %Hidden Layer
end
ym=w'*h; %Output Layer

d_w=0*w;
d_w=(xite*(y-ym))*h;
w = w + d_w +alfa*(w_1 - w_2);
w2 = w_1;
w1=w;

d_b=0*b;
for k=1:5
d_b(k)=(eta*(y-ym))*w(k)*h(k)*(x-c(k))^2/b(k)^3;
end
b = b + d_b +gamma*(b_1 - b_2);

for k=1:5
if b(k)<= 0
    b(k)=0.1;
end
    
end
b2 = b_1;
b1=b;


d_c=0*c;
for k=1:5
d_c(k)=(eta*(y-ym))*w(k)*(x-c(k))/b(k)^2;
end
c = c + d_c +gamma*(c_1 - c_2);

for k=1:5
if abs(c(k))> 100
    c(k)= sign(c(k))*100;
end
end

c2 = c_1;
c1=c;

o=u;
ii=zeros(1);
ii=i+5;

== matlab function position_by_Adaptive_RBF_Attitude_by_supervised_RBFNN/MATLAB Function3 ==
  data: y input; u input; e input; e_d input; ym output; w_1 input; w_2 input; b_1 input; b_2 input; c_1 input; c_2 input; w1 output; w2 output; b1 output; b2 output; c1 output; c2 output; o output; i input; ii output
function [ym,w1,w2,b1,b2,c1,c2,o,ii] =System(y,u,e,e_d,w_1,w_2,b_1,b_2,c_1,c_2,i)
alfa=0.7;
xite=1.79;
eta =0.0000005;
gamma=0.00000001;

 E=[e;e_d];
%Lamda= [0 1 ; -30 -3]; %too slow
%Lamda= [0 1 ; -99 -25]; % vibrating
Lamda= [0 1 ; -5 -9]; %  eig(Lamda)      -0.6993  -14.3007
B=[0;1];
%Q=[0.75 0; 0 0.65];
%Q=[75 0; 0 65];
Q=[7 0; 0 5];
%P = lyap(Lamda',Q);
P=[8.0778    0.7000;    0.7000    0.3556];
%P=[ 7.1500    0.3500;    0.3500    0.1900];
% alfa=0.001;
% xite=0.05;
% eta =0.005;
% gamma=0.0001;


w_1=w_1+zeros(5,1);
w_2=w_2+zeros(5,1);
b_1=b_1+zeros(5,1);
b_2=b_2+zeros(5,1);
c_1=c_1+zeros(5,1);
c_2=c_2+zeros(5,1);
if i == 0
    w=ones(5,1);
    w_1=ones(5,1);
    w_2=ones(5,1)/2;
    b=ones(5,1);
    b=[0.2; 0.2; 0.2; 0.2 ;0.2]*5; %bj
    b_1=b;
    b_2=b;
    c=ones(5,1);
    c=10*[-1.2; -0.5; 0; 0.5 ;1.2]; %cij
    c_1=c;
    c_2=c;
    
      
end

w=w_1;
w1=zeros(5,1); %%%%%%%%%%%%%%%%%%%%  W2
w2=zeros(5,1);
b=b_1;
b1=zeros(5,1);
b2=zeros(5,1);  %%%%%%%%%%%%%%%%%% b2
c=c_1;
c1=zeros(5,1);
c2=zeros(5,1);
x=u; %Input Layer
h=zeros(5,1); %hj
w=w_1;
for j=1:1:5
h(j)=exp(-norm(x-c(j))^2/(2*b(j)^2)); %Hidden Layer
end
ym=w'*h; %Output Layer

d_w=0*w;
d_w= - xite*E'*P*B*h; %%%%%%%%%%%%%%%%%%%%%%%%%%%%%%%%%%%%%%%%%%%%%%%%%%%%%%%%%%%
w = w + d_w + alfa*(w_1 - w_2);
w2 = w_1;
w1=w;

d_b=0*b;
for k=1:5
d_b(k)=(eta*(y-u))*w(k)*h(k)*(x-c(k))^2/b(k)^3;
end
b = b + d_b +gamma*(b_1 - b_2);

for k=1:5
if b(k)<= 0
    b(k)=0.1;
end
    
end
b2 = b_1;
b1=b;


d_c=0*c;
for k=1:5
d_c(k)=(eta*(y-u))*w(k)*(x-c(k))/b(k)^2;
end
c = c + d_c +gamma*(c_1 - c_2);
c2 = c_1;
c1=c;

o=u;
ii=zeros(1);
ii=i+5;

== matlab function position_by_Adaptive_RBF_Attitude_by_supervised_RBFNN/MATLAB Function4 ==
  data: G input; F_est input; phi input; theta input; zdd input; U1 output; ydd input; E input; U2 output
function [U1,U2] = fcn(G,F_est,phi,theta,zdd,ydd,E)
m=1;
g=9.81;
U1=zeros(1);
U2=zeros(1);
%K=[30;3;1];
K=[10;15;0];
u1= (zdd+g)*m/(cos(theta)*cos(phi));

U1=1/G*(-F_est+ydd+K'*E);
U2=K'*E;

%U1=1/G*(-F_est+K'*E);

end
% xdd = f + g u

== matlab function position_by_Adaptive_RBF_Attitude_by_supervised_RBFNN/MATLAB Function5 ==
  data: y input; u input; e input; e_d input; ym output; w_1 input; w_2 input; b_1 input; b_2 input; c_1 input; c_2 input; w1 output; w2 output; b1 output; b2 output; c1 output; c2 output; o output; i input; ii output
function [ym,w1,w2,b1,b2,c1,c2,o,ii] =System(y,u,e,e_d,w_1,w_2,b_1,b_2,c_1,c_2,i)
alfa=0.07;
xite=1.9;
eta =0.0000005;
gamma=0.00000001;
K=[5.5;20;0];
E=[e;e_d];
%Lamda= [0 1 ; -30 -3]; %too slow
%Lamda= [0 1 ; -99 -25]; % vibrating
Lamda= [0 1 ; -5 -9]; %  eig(Lamda)      -0.6993  -14.3007
B=[0;1];
%Q=[0.75 0; 0 0.65];
%Q=[75 0; 0 65];
Q=[7 0; 0 5];
%P = lyap(Lamda',Q);
%P=[8.0778    0.7000;    0.7000    0.3556];
P=[    8.0778    0.7000;    0.7000    0.3556];
% alfa=0.001;
% xite=0.05;
% eta =0.005;
% gamma=0.0001;


w_1=w_1+zeros(5,1);
w_2=w_2+zeros(5,1);
b_1=b_1+zeros(5,1);
b_2=b_2+zeros(5,1);
c_1=c_1+zeros(5,1);
c_2=c_2+zeros(5,1);
if i == 0
    w=ones(5,1);
    w_1=ones(5,1);
    w_2=ones(5,1)/2;
    b=ones(5,1);
    b=[0.2; 0.2; 0.2; 0.2 ;0.2]*5; %bj
    b_1=b;
    b_2=b;
    c=ones(5,1);
    c=10*[-1.2; -0.5; 0; 0.5 ;1.2]; %cij
    c_1=c;
    c_2=c;
    
      
end

w=w_1;
w1=zeros(5,1); %%%%%%%%%%%%%%%%%%%%  W2
w2=zeros(5,1);
b=b_1;
b1=zeros(5,1);
b2=zeros(5,1);  %%%%%%%%%%%%%%%%%% b2
c=c_1;
c1=zeros(5,1);
c2=zeros(5,1);
x=u; %Input Layer
h=zeros(5,1); %hj
w=w_1;
for j=1:1:5
h(j)=exp(-norm(x-c(j))^2/(2*b(j)^2)); %Hidden Layer
end
ym=w'*h; %Output Layer

d_w=0*w;
d_w= - xite*E'*P*B*h; %%%%%%%%%%%%%%%%%%%%%%%%%%%%%%%%%%%%%%%%%%%%%%%%%%%%%%%%%%%
w = w + d_w + alfa*(w_1 - w_2);
w2 = w_1;
w1=w;

d_b=0*b;
for k=1:5
d_b(k)=(eta*(y-u))*w(k)*h(k)*(x-c(k))^2/b(k)^3;
end
b = b + d_b +gamma*(b_1 - b_2);

for k=1:5
if b(k)<= 0
    b(k)=0.1;
end
    
end
b2 = b_1;
b1=b;


d_c=0*c;
for k=1:5
d_c(k)=(eta*(y-u))*w(k)*(x-c(k))/b(k)^2;
end
c = c + d_c +gamma*(c_1 - c_2);
c2 = c_1;
c1=c;

o=u;
ii=zeros(1);
ii=i+5;

== matlab function position_by_Adaptive_RBF_Attitude_by_supervised_RBFNN/Xdd2 ==
  data: phi input; G output; theta input
function G = fcn(phi,theta)
m=1;
g=9.81;
G=(cos(theta)*cos(phi))/m;

== matlab function position_by_Adaptive_RBF_Attitude_by_supervised_RBFNN/Xdd3 ==
  data: fest output
function fest = fcn()

g=9.81;

fest=-g;

== matlab function position_by_Adaptive_RBF_Attitude_by_supervised_RBFNN/MATLAB Function6 ==
  data: G input; F_est input; phi input; theta input; zdd input; U1 output; ydd input; E input; U2 output
function [U1,U2] = fcn(G,F_est,phi,theta,zdd,ydd,E)
m=1;
g=9.81;
U1=zeros(1);
U2=zeros(1);
%K=[10;15;0];
K=[11.3;21;0];
u1= (zdd+g)*m/(cos(theta)*cos(phi));

U1=1/G*(-F_est+ydd+K'*E);
U2=K'*E;

%U1=1/G*(-F_est+K'*E);

end
% xdd = f + g u

== matlab function position_by_Adaptive_RBF_Attitude_by_supervised_RBFNN/Xdd1 ==
  data: phi input; G output; theta input; ksi input
function G = fcn(phi,theta, ksi)
m=1;
g=9.81;
G=(sin(ksi)*sin(phi)+cos(ksi)*sin(theta)*cos(phi))/m;
G=1;

== matlab function position_by_Adaptive_RBF_Attitude_by_supervised_RBFNN/Xdd4 ==
  data: fest output
function fest = fcn()

g=9.81;

fest=0;
